simulink model "Project"  (R2018a)
settings: Solver=VariableStepAuto  StartTime=0.0  StopTime=10.0  RelTol=1e-3
libraries: legoev3lib x2
settings Model: Creator=Lenovo  LastModifiedBy=Lenovo

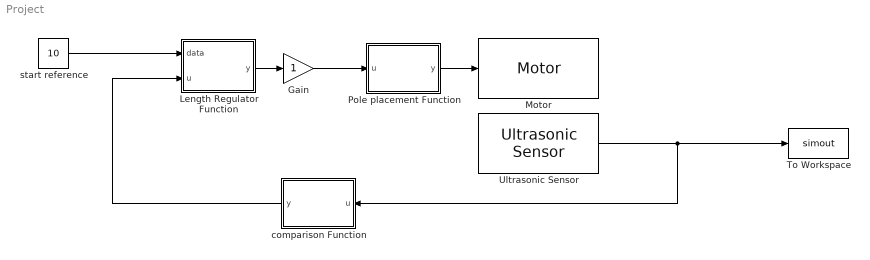
== system Project ==
  Gain : Gain
  Length Regulator Function : MATLAB Function  TreatAsAtomicUnit=on
  Motor : legoev3lib/Motor  sportNumber=A  sstopAction=Brake
  Pole placement Function : MATLAB Function  TreatAsAtomicUnit=on
  To Workspace : ToWorkspace  VariableName=simout  SaveFormat=Timeseries  SampleTime=-1
  Ultrasonic Sensor : legoev3lib/Ultrasonic Sensor  PortNumber=1  sampleTime=0.1
      settings: SourceProductName=Simulink Support Package for LEGO MINDSTORMS EV3 Hardware  SourceProductBaseCode=LEGOEV3
  comparison Function : MATLAB Function  TreatAsAtomicUnit=on
  start reference : Constant  Value=10
  wires:
  Length Regulator Function/1(y) -> Gain/1
  Ultrasonic Sensor/1 -> comparison Function/1(u), To Workspace/1
  start reference/1 -> Length Regulator Function/1(data)
  comparison Function/1(y) -> Length Regulator Function/2(u)
  Gain/1 -> Pole placement Function/1(u)
  Pole placement Function/1(y) -> Motor/1

== matlab function Project/comparison Function ==
  data: u input; y output
function y = fcn(u)

if(u>40)
y = 40;
else
y = u;
    
end

== matlab function Project/Length Regulator Function ==
  data: data input; u input; y output
function y = fcn(data, u)
x = data;
y = x-u;

== matlab function Project/Pole placement Function ==
  data: u input; y output
function y = fcn(u)

y = u;
